simulink model "EZE4sRStEnCtrl"  (R2018b)
settings: Solver=FixedStepDiscrete  StartTime=0.0  StopTime=10.0  FixedStep=0.01  RelTol=1e-3
undefined symbols (not defined in the file or in its folder): data, SecRwRtStBkReclnEn_Clear, SecRwRtStBkReclnEn_Set, SecRwRtStFwdBkwdEn_Clear, SecRwRtStFwdBkwdEn_Set, SecRwRtStHdrstFwdBkwdEn_Clear, SecRwRtStHdrstFwdBkwdEn_Set, SecRwRtStHdrstUpwdDnwdEn_Clear, SecRwRtStHdrstUpwdDnwdEn_Set
libraries: simulink x1
settings Model: ModifiedHistory=2023.8.1 V2.0.0 CR421790 增加模式21-26  Creator=sn2xws  LastModifiedBy=sn2xws
settings DataIOCC: SaveFormat=StructureWithTime
settings OptimizationCC: DefaultParameterBehavior=Inlined  EnhancedBackFolding=on  PassReuseOutputArgsAs=Individual arguments  ZeroExternalMemoryAtStartup=off  ZeroInternalMemoryAtStartup=off  OptimizeBlockOrder=speed  DifferentSizesBufferReuse=on  OptimizationCustomize=off
settings DebuggingCC: ParameterTunabilityLossMsg=error
settings SFSimCC: MATLABDynamicMemAlloc=off
settings RTWCC: SystemTargetFile=autosar.tlc  GenCodeOnly=on  TemplateMakefile=ert_default_tmf  Description=AUTOSAR  GenerateReport=on  IncludeHyperlinkInReport=on  LaunchReport=on  GenerateTraceInfo=on  GenerateTraceReport=on  GenerateTraceReportSl=on  GenerateTraceReportSf=on  GenerateTraceReportEml=on  GenerateCodeMetricsReport=on
settings CodeAppCC: ForceParamTrailComments=on  IgnoreCustomStorageClasses=off  OperatorAnnotations=on  SimulinkDataObjDesc=on  SFDataObjDesc=on  InsertBlockDesc=on
settings STFCustomTargetCC: TargetLangStandard=C99 (ISO)  MultiwordLength=256  ParMdlRefBuildCompliant=on  CompOptLevelCompliant=on  IncludeMdlTerminateFcn=off  CombineOutputUpdateFcns=on  SuppressErrorStatus=on  ERTCustomFileBanners=on  SupportNonFinite=off  SupportComplex=off  SupportContinuousTime=off  SupportNonInlinedSFcns=off  RemoveResetFunc=on  MATLABClassNameForMDSCustomization=Simulink.SoftwareTarget.ERTCustomization  AutosarCompliant=on  UseToolchainInfoCompliant=on  LookupTableObjectStructAxisOrder=2,1,3,4,...  LUTObjectStructOrderEvenSpacing=Size,Table,Breakpoints  SystemTargetFile=autosar.tlc
settings ERTTargetCC: TargetLangStandard=C99 (ISO)  ConcurrentExecutionCompliant=off  IncludeMdlTerminateFcn=off  SuppressErrorStatus=on  SupportNonFinite=off  SupportComplex=off  ModelStepFunctionPrototypeControlCompliant=off  CPPClassGenCompliant=off  AutosarCompliant=on  LookupTableObjectStructAxisOrder=2,1,3,4,...  LUTObjectStructOrderEvenSpacing=Size,Table,Breakpoints  InlinedParameterPlacement=NonHierarchical  ERTCustomFileTemplate=example_file_process.tlc  ERTFilePackagingFormat=Compact

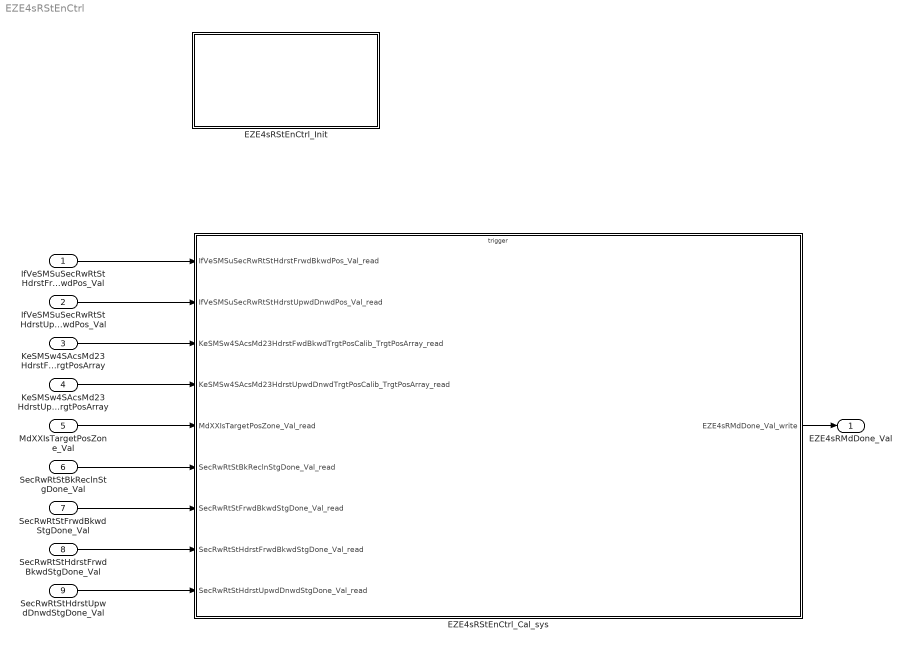
== system EZE4sRStEnCtrl ==
  IfVeSMSuSecRwRtStHdrstFrwdBkwdPos_Val : Inport  OutDataTypeStr=uint16  PortDimensions=1
  IfVeSMSuSecRwRtStHdrstUpwdDnwdPos_Val : Inport  Port=2  OutDataTypeStr=uint16  PortDimensions=1
  KeSMSw4SAcsMd23HdrstFwdBkwdTrgtPosCalib_TrgtPosArray : Inport  Description=|  Port=3  OutDataTypeStr=uint16  PortDimensions=3
      | 0:Pos
      | 1:Max
      | 2:Min
  KeSMSw4SAcsMd23HdrstUpwdDnwdTrgtPosCalib_TrgtPosArray : Inport  Description=|  Port=4  OutDataTypeStr=uint16  PortDimensions=3
      | 0:Pos
      | 1:Max
      | 2:Min
  MdXXIsTargetPosZone_Val : Inport  Port=5  OutDataTypeStr=uint32  PortDimensions=1
  SecRwRtStBkReclnStgDone_Val : Inport  Port=6  OutDataTypeStr=boolean  PortDimensions=1
  SecRwRtStFrwdBkwdStgDone_Val : Inport  Port=7  OutDataTypeStr=boolean  PortDimensions=1
  SecRwRtStHdrstFrwdBkwdStgDone_Val : Inport  Port=8  OutDataTypeStr=boolean  PortDimensions=1
  SecRwRtStHdrstUpwdDnwdStgDone_Val : Inport  Port=9  OutDataTypeStr=boolean  PortDimensions=1
  EZE4sRStEnCtrl_Cal_sys : Subsystem
  EZE4sRStEnCtrl_Init : Subsystem
  EZE4sRMdDone_Val : Outport  OutDataTypeStr=uint8  PortDimensions=1
  wires:
  IfVeSMSuSecRwRtStHdrstFrwdBkwdPos_Val/1 -> EZE4sRStEnCtrl_Cal_sys/1(IfVeSMSuSecRwRtStHdrstFrwdBkwdPos_Val_read)
  IfVeSMSuSecRwRtStHdrstUpwdDnwdPos_Val/1 -> EZE4sRStEnCtrl_Cal_sys/2(IfVeSMSuSecRwRtStHdrstUpwdDnwdPos_Val_read)
  KeSMSw4SAcsMd23HdrstFwdBkwdTrgtPosCalib_TrgtPosArray/1 -> EZE4sRStEnCtrl_Cal_sys/3(KeSMSw4SAcsMd23HdrstFwdBkwdTrgtPosCalib_TrgtPosArray_read)
  KeSMSw4SAcsMd23HdrstUpwdDnwdTrgtPosCalib_TrgtPosArray/1 -> EZE4sRStEnCtrl_Cal_sys/4(KeSMSw4SAcsMd23HdrstUpwdDnwdTrgtPosCalib_TrgtPosArray_read)
  MdXXIsTargetPosZone_Val/1 -> EZE4sRStEnCtrl_Cal_sys/5(MdXXIsTargetPosZone_Val_read)
  SecRwRtStBkReclnStgDone_Val/1 -> EZE4sRStEnCtrl_Cal_sys/6(SecRwRtStBkReclnStgDone_Val_read)
  SecRwRtStFrwdBkwdStgDone_Val/1 -> EZE4sRStEnCtrl_Cal_sys/7(SecRwRtStFrwdBkwdStgDone_Val_read)
  SecRwRtStHdrstFrwdBkwdStgDone_Val/1 -> EZE4sRStEnCtrl_Cal_sys/8(SecRwRtStHdrstFrwdBkwdStgDone_Val_read)
  SecRwRtStHdrstUpwdDnwdStgDone_Val/1 -> EZE4sRStEnCtrl_Cal_sys/9(SecRwRtStHdrstUpwdDnwdStgDone_Val_read)
  EZE4sRStEnCtrl_Cal_sys/1(EZE4sRMdDone_Val_write) -> EZE4sRMdDone_Val/1

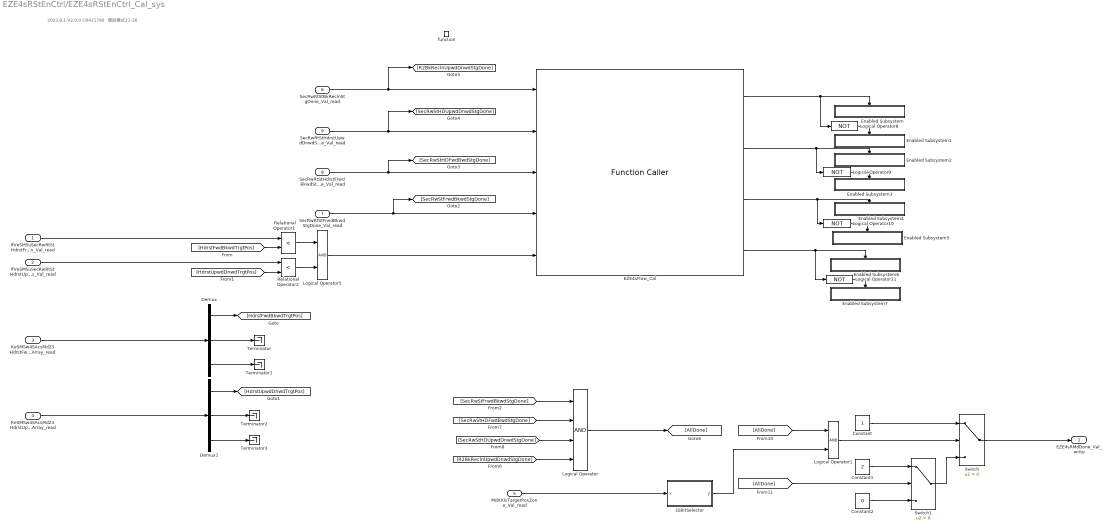
== system EZE4sRStEnCtrl/EZE4sRStEnCtrl_Cal_sys ==
  note: 2023.8.1 V2.0.0 CR421790 增加模式21-26
  IfVeSMSuSecRwRtStHdrstFrwdBkwdPos_Val_read : Inport
  IfVeSMSuSecRwRtStHdrstUpwdDnwdPos_Val_read : Inport  Port=2
  KeSMSw4SAcsMd23HdrstFwdBkwdTrgtPosCalib_TrgtPosArray_read : Inport  Port=3
  KeSMSw4SAcsMd23HdrstUpwdDnwdTrgtPosCalib_TrgtPosArray_read : Inport  Port=4
  MdXXIsTargetPosZone_Val_read : Inport  Port=5
  SecRwRtStBkReclnStgDone_Val_read : Inport  Port=6
  SecRwRtStFrwdBkwdStgDone_Val_read : Inport  Port=7
  SecRwRtStHdrstFrwdBkwdStgDone_Val_read : Inport  Port=8
  SecRwRtStHdrstUpwdDnwdStgDone_Val_read : Inport  Port=9
  function : TriggerPort  TriggerType=function-call  IsSimulinkFunction=on  FunctionName=EZE4sRStEnCtrl_Cal  VariantControl=(inherit)
  32BitSelector : Subsystem  mask(32 Bit Selector){BitNum=22}
      mask prompts: BitNum "Select Bit Number"
      mask help: Allows selection of a particular bit (0-31) out of a packed word up to 32 bits long. Output will be true if the bit number selected via the mask parameter is equal to one.
      mask TypeOptions BitNum: 0 | 1 | 2 | 3 | 4 | 5 | 6 | 7 | 8 | 9 | 10 | 11 | 12 | 13 | 14 | 15 | 16 | 17 | 18 | 19 | 20 | 21 | 22 | 23 | 24 | 25 | 26 | 27 | 28 | 29 | 30 | 31
      mask Display:
      | text(0.5, 0.8,'BIT','horizontalAlignment','center')
      | text(0.5, 0.5,'SELECTOR','horizontalAlignment','center')
      | text(0.5, 0.2,['-- Bit ',char(get_param(gcb,'BitNum')),' --'],'horizontalAlignment','center')
  Constant : Constant  OutDataTypeStr=uint8
  Constant1 : Constant  Value=2  OutDataTypeStr=uint8
  Constant2 : Constant  Value=0  OutDataTypeStr=uint8
  Demux : Demux  Outputs=3
  Demux1 : Demux  Outputs=3
  EZE4sFlow_Cal : FunctionCaller  FunctionPrototype=[BkReclnEn,HdrstUpwdEn,HdrstFrwdEn,SecRwStFrwdBkwdEn] = EZE4sFlow_Cal(BkReclnStgDone,HdrstUpwdDnwdStgDone,HdrstFrwdBkwdStgDone,SecRwStFrwdBkwdStgDone,Chkhdflg)  InputArgumentSpecifications=boolean(true), boolean(true), boolean(true), boolean(true), boolean(true)  OutputArgumentSpecifications=boolean(true), boolean(true), boolean(true), boolean(true)
  Enabled Subsystem : Subsystem  TreatAsAtomicUnit=on
  Enabled Subsystem1 : Subsystem  TreatAsAtomicUnit=on
  Enabled Subsystem2 : Subsystem  TreatAsAtomicUnit=on
  Enabled Subsystem3 : Subsystem  TreatAsAtomicUnit=on
  Enabled Subsystem4 : Subsystem  TreatAsAtomicUnit=on
  Enabled Subsystem5 : Subsystem  TreatAsAtomicUnit=on
  Enabled Subsystem6 : Subsystem  TreatAsAtomicUnit=on
  Enabled Subsystem7 : Subsystem  TreatAsAtomicUnit=on
  Logical Operator : Logic  Inputs=4  AllPortsSameDT=off  OutDataTypeStr=boolean
  Logical Operator1 : Logic  AllPortsSameDT=off  OutDataTypeStr=boolean
  Logical Operator{8..11} (4 alike) : Logic  Operator=NOT  AllPortsSameDT=off  OutDataTypeStr=boolean
  Logical Operator5 : Logic  AllPortsSameDT=off  OutDataTypeStr=boolean
  Relational Operator1 : RelationalOperator  Operator=<  OutDataTypeStr=boolean  RndMeth=Simplest
  Relational Operator2 : RelationalOperator  Operator=<  OutDataTypeStr=boolean  RndMeth=Simplest
  Switch : Switch  Criteria=u2 > Threshold
  Switch1 : Switch  Criteria=u2 > Threshold
  Terminator{,1..3} (4 alike) : Terminator
  EZE4sRMdDone_Val_write : Outport
      settings: EnsureOutportIsVirtual=on
  wires:
  SecRwRtStBkReclnStgDone_Val_read/1 -> [R2BkReclnUpwdDnwdStgDone], EZE4sFlow_Cal/1
  SecRwRtStHdrstUpwdDnwdStgDone_Val_read/1 -> [SecRwStHDUpwdDnwdStgDone], EZE4sFlow_Cal/2
  SecRwRtStHdrstFrwdBkwdStgDone_Val_read/1 -> [SecRwStHDFwdBwdStgDone], EZE4sFlow_Cal/3
  SecRwRtStFrwdBkwdStgDone_Val_read/1 -> [SecRwStFrwdBkwdStgDone], EZE4sFlow_Cal/4
  Relational Operator2/1 -> Logical Operator5/2
  [HdrstFwdBkwdTrgtPos] -> Relational Operator1/2
  IfVeSMSuSecRwRtStHdrstFrwdBkwdPos_Val_read/1 -> Relational Operator1/1
  Logical Operator5/1 -> EZE4sFlow_Cal/5
  Relational Operator1/1 -> Logical Operator5/1
  IfVeSMSuSecRwRtStHdrstUpwdDnwdPos_Val_read/1 -> Relational Operator2/1
  [HdrstUpwdDnwdTrgtPos] -> Relational Operator2/2
  Demux1/1 -> [HdrstUpwdDnwdTrgtPos]
  Demux/2 -> Terminator/1
  Demux/1 -> [HdrstFwdBkwdTrgtPos]
  KeSMSw4SAcsMd23HdrstUpwdDnwdTrgtPosCalib_TrgtPosArray_read/1 -> Demux1/1
  KeSMSw4SAcsMd23HdrstFwdBkwdTrgtPosCalib_TrgtPosArray_read/1 -> Demux/1
  Demux1/3 -> Terminator3/1
  Demux1/2 -> Terminator2/1
  Demux/3 -> Terminator1/1
  [R2BkReclnUpwdDnwdStgDone] -> Logical Operator/4
  Logical Operator/1 -> [AllDone]
  [SecRwStHDFwdBwdStgDone] -> Logical Operator/2
  [SecRwStHDUpwdDnwdStgDone] -> Logical Operator/3
  [SecRwStFrwdBkwdStgDone] -> Logical Operator/1
  Switch1/1 -> Switch/3
  Constant/1 -> Switch/1
  Switch/1 -> EZE4sRMdDone_Val_write/1
  Constant2/1 -> Switch1/3
  MdXXIsTargetPosZone_Val_read/1 -> 32BitSelector/1(x)
  Logical Operator1/1 -> Switch/2
  [AllDone] -> Switch1/2
  [AllDone] -> Logical Operator1/1
  Constant1/1 -> Switch1/1
  32BitSelector/1(y) -> Logical Operator1/2
  EZE4sFlow_Cal/4 -> Logical Operator11/1, Enabled Subsystem6/Enable
  Logical Operator10/1 -> Enabled Subsystem5/Enable
  Logical Operator9/1 -> Enabled Subsystem3/Enable
  Logical Operator11/1 -> Enabled Subsystem7/Enable
  Logical Operator8/1 -> Enabled Subsystem1/Enable
  EZE4sFlow_Cal/3 -> Logical Operator10/1, Enabled Subsystem4/Enable
  EZE4sFlow_Cal/1 -> Logical Operator8/1, Enabled Subsystem/Enable
  EZE4sFlow_Cal/2 -> Logical Operator9/1, Enabled Subsystem2/Enable

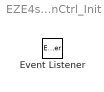
== system EZE4sRStEnCtrl/EZE4sRStEnCtrl_Init ==
  Event Listener : EventListener  EventName=reset

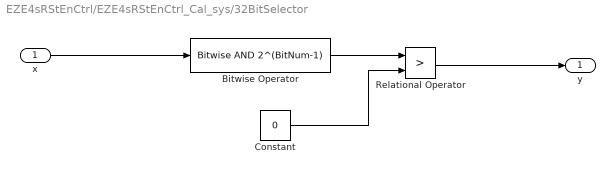
== system EZE4sRStEnCtrl/EZE4sRStEnCtrl_Cal_sys/32BitSelector ==
  x : Inport
  Bitwise Operator : simulink/Logic and Bit Operations/Bitwise Operator  logicop=AND  UseBitMask=on  BitMask=2^(BitNum-1)  BitMaskRealWorld=Stored Integer
  Constant : Constant  Value=0  OutDataTypeStr=uint32
  Relational Operator : RelationalOperator  Operator=>  OutDataTypeStr=boolean  RndMeth=Simplest
  y : Outport
  wires:
  Relational Operator/1 -> y/1
  Constant/1 -> Relational Operator/2
  x/1 -> Bitwise Operator/1
  Bitwise Operator/1 -> Relational Operator/1

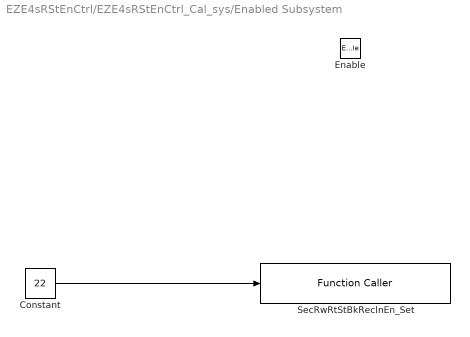
== system EZE4sRStEnCtrl/EZE4sRStEnCtrl_Cal_sys/Enabled Subsystem ==
  Enable : EnablePort
  Constant : Constant  Value=22  OutDataTypeStr=uint8
  SecRwRtStBkReclnEn_Set : FunctionCaller  FunctionPrototype=SecRwRtStBkReclnEn_Set(data)  InputArgumentSpecifications=uint8(1)
  wires:
  Constant/1 -> SecRwRtStBkReclnEn_Set/1

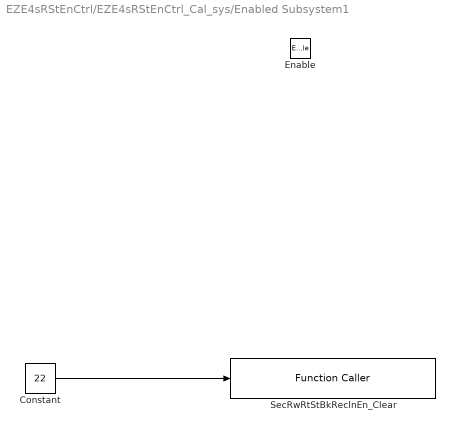
== system EZE4sRStEnCtrl/EZE4sRStEnCtrl_Cal_sys/Enabled Subsystem1 ==
  Enable : EnablePort
  Constant : Constant  Value=22  OutDataTypeStr=uint8
  SecRwRtStBkReclnEn_Clear : FunctionCaller  FunctionPrototype=SecRwRtStBkReclnEn_Clear(data)  InputArgumentSpecifications=uint8(1)
  wires:
  Constant/1 -> SecRwRtStBkReclnEn_Clear/1

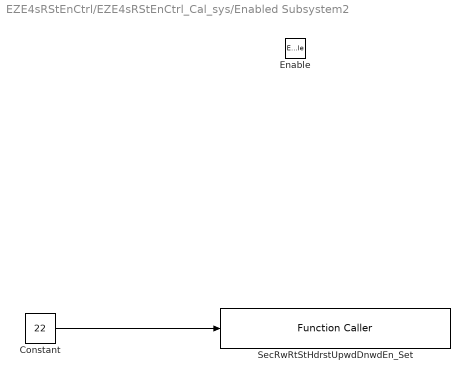
== system EZE4sRStEnCtrl/EZE4sRStEnCtrl_Cal_sys/Enabled Subsystem2 ==
  Enable : EnablePort
  Constant : Constant  Value=22  OutDataTypeStr=uint8
  SecRwRtStHdrstUpwdDnwdEn_Set : FunctionCaller  FunctionPrototype=SecRwRtStHdrstUpwdDnwdEn_Set(data)  InputArgumentSpecifications=uint8(1)
  wires:
  Constant/1 -> SecRwRtStHdrstUpwdDnwdEn_Set/1

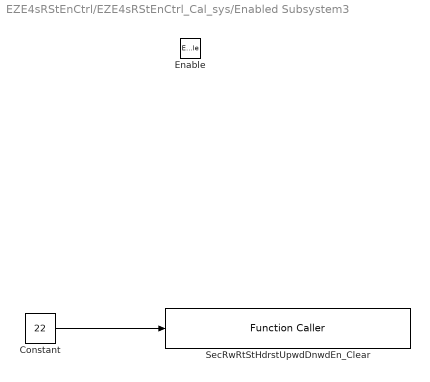
== system EZE4sRStEnCtrl/EZE4sRStEnCtrl_Cal_sys/Enabled Subsystem3 ==
  Enable : EnablePort
  Constant : Constant  Value=22  OutDataTypeStr=uint8
  SecRwRtStHdrstUpwdDnwdEn_Clear : FunctionCaller  FunctionPrototype=SecRwRtStHdrstUpwdDnwdEn_Clear(data)  InputArgumentSpecifications=uint8(1)
  wires:
  Constant/1 -> SecRwRtStHdrstUpwdDnwdEn_Clear/1

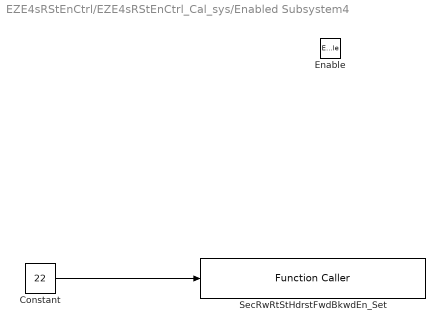
== system EZE4sRStEnCtrl/EZE4sRStEnCtrl_Cal_sys/Enabled Subsystem4 ==
  Enable : EnablePort
  Constant : Constant  Value=22  OutDataTypeStr=uint8
  SecRwRtStHdrstFwdBkwdEn_Set : FunctionCaller  FunctionPrototype=SecRwRtStHdrstFwdBkwdEn_Set(data)  InputArgumentSpecifications=uint8(1)
  wires:
  Constant/1 -> SecRwRtStHdrstFwdBkwdEn_Set/1

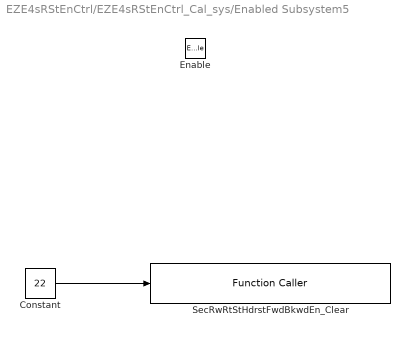
== system EZE4sRStEnCtrl/EZE4sRStEnCtrl_Cal_sys/Enabled Subsystem5 ==
  Enable : EnablePort
  Constant : Constant  Value=22  OutDataTypeStr=uint8
  SecRwRtStHdrstFwdBkwdEn_Clear : FunctionCaller  FunctionPrototype=SecRwRtStHdrstFwdBkwdEn_Clear(data)  InputArgumentSpecifications=uint8(1)
  wires:
  Constant/1 -> SecRwRtStHdrstFwdBkwdEn_Clear/1

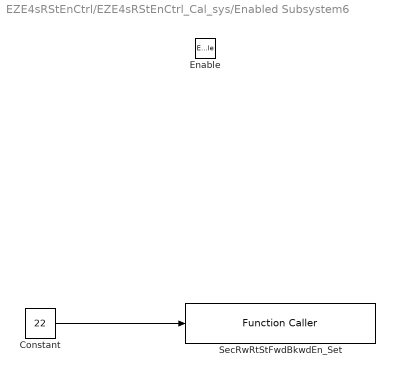
== system EZE4sRStEnCtrl/EZE4sRStEnCtrl_Cal_sys/Enabled Subsystem6 ==
  Enable : EnablePort
  Constant : Constant  Value=22  OutDataTypeStr=uint8
  SecRwRtStFwdBkwdEn_Set : FunctionCaller  FunctionPrototype=SecRwRtStFwdBkwdEn_Set(data)  InputArgumentSpecifications=uint8(1)
  wires:
  Constant/1 -> SecRwRtStFwdBkwdEn_Set/1

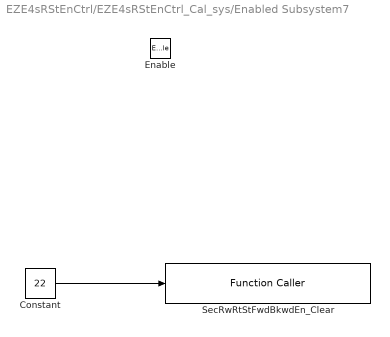
== system EZE4sRStEnCtrl/EZE4sRStEnCtrl_Cal_sys/Enabled Subsystem7 ==
  Enable : EnablePort
  Constant : Constant  Value=22  OutDataTypeStr=uint8
  SecRwRtStFwdBkwdEn_Clear : FunctionCaller  FunctionPrototype=SecRwRtStFwdBkwdEn_Clear(data)  InputArgumentSpecifications=uint8(1)
  wires:
  Constant/1 -> SecRwRtStFwdBkwdEn_Clear/1
